simulink library "All_Sensors_Working"  (R2020a)
settings: Solver=ode45  StartTime=0.0  StopTime=10.0  RelTol=1e-3  EnableMultiTasking=on
undefined symbols (not defined in the file): CR
libraries: simulink x10
settings Model: Creator=aldernl  LastModifiedBy=Harjot
settings DataIOCC: LimitDataPoints=on
settings OptimizationCC: LifeSpan=inf
settings DebuggingCC: AllowSymbolicDim=off  SFUnexpectedBacktrackingDiag=warning  SFNoUnconditionalDefaultTransitionDiag=warning  ArithmeticOperatorsInVariantConditions=warning
settings SFSimCC: SimUseLocalCustomCode=off  CustomCodeUndefinedFunction=UseInterfaceOnly
settings RTWCC: RTWUseLocalCustomCode=off
settings CodeAppCC: StateflowObjectComments=on
settings GRTTargetCC: TargetLangStandard=C89/C90 (ANSI)
settings ConfigComp: CovMetricSettings=dw  CovHtmlReporting=on  CovSaveCumulativeToWorkspaceVar=on  CovSaveSingleToWorkspaceVar=on  CovExternalEMLEnable=off

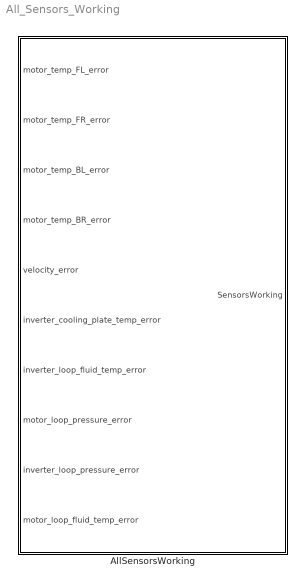
== system All_Sensors_Working ==
  AllSensorsWorking : Subsystem

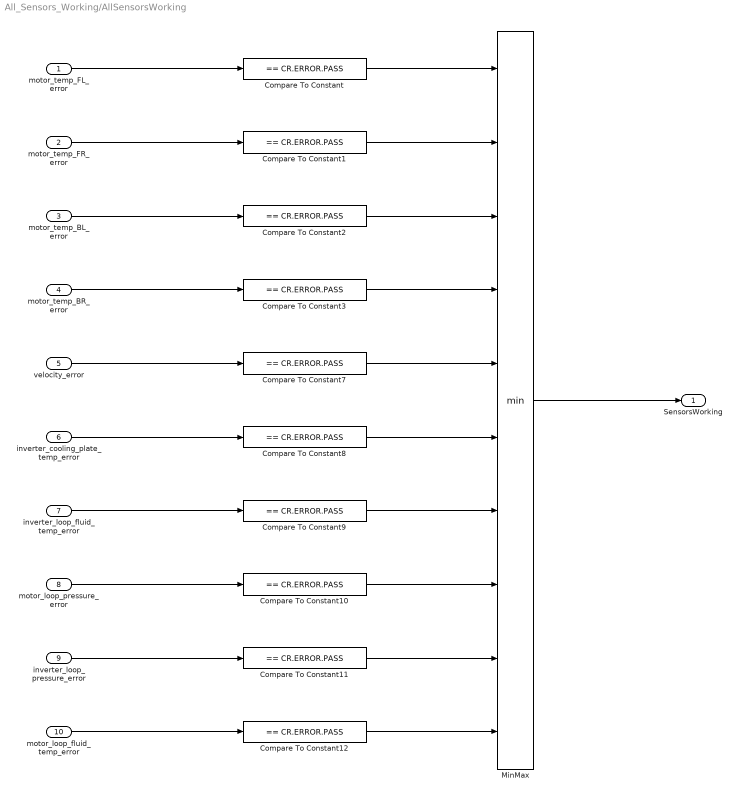
== system All_Sensors_Working/AllSensorsWorking ==
  motor_temp_FL_error : Inport  OutDataTypeStr=double  PortDimensions=1
  motor_temp_FR_error : Inport  Port=2  OutDataTypeStr=double  PortDimensions=1
  motor_temp_BL_error : Inport  Port=3  OutDataTypeStr=double  PortDimensions=1
  motor_temp_BR_error : Inport  Port=4  OutDataTypeStr=double  PortDimensions=1
  velocity_error : Inport  Port=5  OutDataTypeStr=double  PortDimensions=1
  inverter_cooling_plate_temp_error : Inport  Port=6  OutDataTypeStr=double  PortDimensions=1
  inverter_loop_fluid_temp_error : Inport  Port=7  OutDataTypeStr=double  PortDimensions=1
  motor_loop_pressure_error : Inport  Port=8  OutDataTypeStr=double  PortDimensions=1
  inverter_loop_pressure_error : Inport  Port=9  OutDataTypeStr=double  PortDimensions=1
  motor_loop_fluid_temp_error : Inport  Port=10  OutDataTypeStr=double  PortDimensions=1
  Compare To Constant{,1..3,7..12} (10 alike) : simulink/Logic and Bit Operations/Compare To Constant  relop===  const=CR.ERROR.PASS  OutDataTypeStr=uint8
  MinMax : MinMax  Inputs=10  OutDataTypeStr=double
  SensorsWorking : Outport  VectorParamsAs1DForOutWhenUnconnected=off
  wires:
  motor_loop_fluid_temp_error/1 -> Compare To Constant12/1
  Compare To Constant12/1 -> MinMax/10
  Compare To Constant11/1 -> MinMax/9
  Compare To Constant10/1 -> MinMax/8
  Compare To Constant9/1 -> MinMax/7
  Compare To Constant8/1 -> MinMax/6
  Compare To Constant7/1 -> MinMax/5
  inverter_loop_pressure_error/1 -> Compare To Constant11/1
  motor_loop_pressure_error/1 -> Compare To Constant10/1
  inverter_loop_fluid_temp_error/1 -> Compare To Constant9/1
  inverter_cooling_plate_temp_error/1 -> Compare To Constant8/1
  velocity_error/1 -> Compare To Constant7/1
  motor_temp_FL_error/1 -> Compare To Constant/1
  motor_temp_FR_error/1 -> Compare To Constant1/1
  motor_temp_BL_error/1 -> Compare To Constant2/1
  motor_temp_BR_error/1 -> Compare To Constant3/1
  MinMax/1 -> SensorsWorking/1
  Compare To Constant1/1 -> MinMax/2
  Compare To Constant2/1 -> MinMax/3
  Compare To Constant3/1 -> MinMax/4
  Compare To Constant/1 -> MinMax/1
